simulink model "state_machine_by_cod_1_sm_master"  (R2021b)
settings: Solver=ode4  StartTime=0.0  StopTime=inf  FixedStep=0.001  RelTol=1e-3  EnableMultiTasking=on
model workspace (MATLAB code in the model file):
  | addpath src\model
  | addpath src\utils
libraries: opal_lib x3
Description:
  | Model of a simple control system for use iin training.
settings Model: Creator=Paul Baracos  LastModifiedBy=andrerangel
settings SolverCC: AlgebraicLoopSolver=TrustRegion
settings DataIOCC: LimitDataPoints=on  SaveFormat=Array  SignalLoggingSaveFormat=ModelDataLogs  SaveOutput=off  SaveTime=off  ReturnWorkspaceOutputs=off  SignalLoggingName=sigsOut
settings OptimizationCC: BlockReduction=off  BooleanDataType=off  OptimizeBlockIOStorage=off  BufferReuse=off  ExpressionFolding=off  LocalBlockOutputs=off  InitFltsAndDblsToZero=on  LifeSpan=inf
settings DebuggingCC: SaveWithParameterizedLinksMsg=none  UnderspecifiedInitializationDetection=Classic  MergeDetectMultiDrivingBlocksExec=none  SignalResolutionControl=TryResolveAllWithWarning  MultiTaskDSMMsg=warning  MultiTaskCondExecSysMsg=none  FcnCallInpInsideContextMsg=warning  SFUnexpectedBacktrackingDiag=warning  SFNoUnconditionalDefaultTransitionDiag=warning  SFExecutionAtInitializationDiag=none  SFMachineParentedDataDiag=warning  ArithmeticOperatorsInVariantConditions=warning
settings HardwareCC: ProdBitPerPointer=32  ProdBitPerSizeT=32  ProdBitPerPtrDiffT=32  ProdLargestAtomicFloat=None  ProdIntDivRoundTo=Undefined  ProdEndianess=Unspecified  ProdWordSize=32  ProdHWDeviceType=32-bit Generic  TargetUnknown=on
settings ModelReferenceCC: PropagateSignalLabelsOutOfModel=off
settings SFSimCC: SimUseLocalCustomCode=off  CustomCodeUndefinedFunction=UseInterfaceOnly
settings RTWCC: GenCodeOnly=on  RTWUseLocalCustomCode=off
settings CodeAppCC: StateflowObjectComments=on
settings GRTTargetCC: TargetFcnLib=ansi_tfl_tmw.mat  TargetLangStandard=C89/C90 (ANSI)  CombineOutputUpdateFcns=off  GRTInterface=on
settings ConfigComp: CovMetricSettings=dw  CovSaveCumulativeToWorkspaceVar=on  CovSaveSingleToWorkspaceVar=on  CovExternalEMLEnable=off

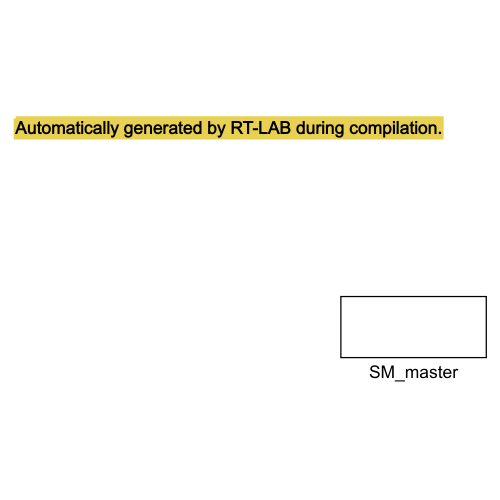
[thumbnail: Simulink's stored preview of the top-level diagram]
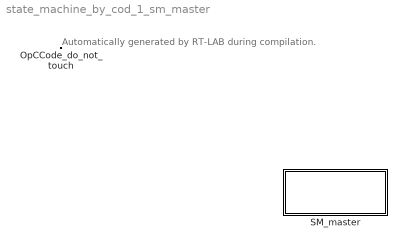
== system state_machine_by_cod_1_sm_master ==
  note: Automatically generated by RT-LAB during compilation.
  OpCCode_do_not_touch : opal_lib/Communication/OpCCode  SystemSampleTime=-1  VariantActivationTime=update diagram  Latency=0  AutoFrameSizeCalculation=off
  SM_master : Subsystem

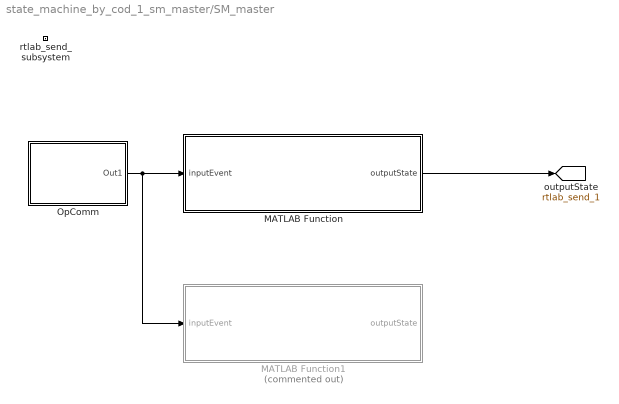
== system state_machine_by_cod_1_sm_master/SM_master ==
  MATLAB Function : MATLAB Function  TreatAsAtomicUnit=on
  MATLAB Function1 : MATLAB Function  Commented=on  TreatAsAtomicUnit=on
  OpComm : Subsystem
      mask init:
      | opmaskdisplay('maskdisplay_block',gcb,'disp(''OpComm'')');
      mask Display:
      | patch([0 0.5 0.7 0],[1 1 0 0],[0.7 0.75 0.9]);
      | patch([1 0.53 0.73 1],[1 1 0 0],[1 0.8 0.7]);
      | plot([0 0 1 1 0],[0 1 1 0 0]);
      | disp('OpComm')
  rtlab_send_subsystem : Subsystem  Priority=-100
      mask Display: text(0,0,'');
  tag scope: rtlab_send_1=global
  wires:
  MATLAB Function/1(outputState) -> [rtlab_send_1]
  OpComm/1(Out1) -> MATLAB Function1/1(inputEvent), MATLAB Function/1(inputEvent)

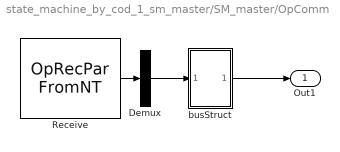
== system state_machine_by_cod_1_sm_master/SM_master/OpComm ==
  Demux : Demux  Outputs=[1]
  Receive : opal_lib/Communication/OpRecPar FromNT  Data_width=1  InitialConditions=3
  busStruct : Subsystem
  Out1 : Outport
  wires:
  Demux/1 -> busStruct/1(In1)
  busStruct/1(Out1) -> Out1/1
  Receive/1 -> Demux/1

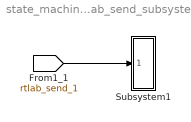
== system state_machine_by_cod_1_sm_master/SM_master/rtlab_send_subsystem ==
  Subsystem1 : Subsystem
  wires:
  [rtlab_send_1] -> Subsystem1/1(In1)

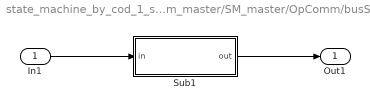
== system state_machine_by_cod_1_sm_master/SM_master/OpComm/busStruct ==
  In1 : Inport
  Sub1 : Subsystem
  Out1 : Outport
  wires:
  Sub1/1(out) -> Out1/1
  In1/1 -> Sub1/1(in)

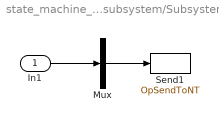
== system state_machine_by_cod_1_sm_master/SM_master/rtlab_send_subsystem/Subsystem1 ==
  In1 : Inport
  Mux : Mux  Inputs=1
  Send1 : opal_lib/Communication/OpSendToNT  Acqu_group=1
  wires:
  Mux/1 -> Send1/1
  In1/1 -> Mux/1

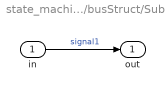
== system state_machine_by_cod_1_sm_master/SM_master/OpComm/busStruct/Sub1 ==
  in : Inport
  out : Outport
  wires:
  in/1 -> out/1  "signal1"

== matlab function state_machine_by_cod_1_sm_master/SM_master/MATLAB Function ==
  data: inputEvent input; outputState output size=[1 1]
function outputState   = stateMachineFcn(inputEvent)
% Example of a State Machine with 3 states.
persistent stateMachine

if (isempty(stateMachine))
    
    % Create the states with the State Class.
    s0 = State(0, 's0', [1,0,1,1,1]);
    s1 = State(1, 's1', [1,1,0,1,1]);
    s2 = State(2, 's2', [1,0,1,1,1]);

    % Group it in a cell array.
    statesArray = {s0, s1, s2};

    % Transitions matrix where each line represents a transition: 
    % event 2 makes a transitions from state 0 to 2 is represented as 
    % [0 2 1]
    transitions = [0, 1 0; 0, 2, 1; 1, 3, 0; 1, 4, 2; 2, 5, 1; 2, 1, 0];

    % Array with the number of the events.
    eventsArray = [1 2 3 4 5];
    stateMachine = StateMachine(statesArray, transitions, eventsArray);
end

stateMachine.inputEvent = inputEvent;
outputState = double(stateMachine.currentState.number);

%activeEvents = stateMachine.currentState.activeEvents;

== matlab function state_machine_by_cod_1_sm_master/SM_master/MATLAB Function1 ==
  data: inputEvent input; outputState output size=[1 1]
function outputState   = stateMachineDebug(inputEvent)
% Example of a State Machine with 3 states.
persistent stateMachine
persistent statesArray
persistent transitions
persistent stateNumber
persistent stateIndex
persistent numberOfStates
persistent eventsArray

if (isempty(stateMachine))
    stateMachine = 1;
    % Create the states with the State Class.
    s0 = State(0, 's0', [1,0,1,1,1]);
    s1 = State(1, 's1', [1,1,0,1,1]);
    s2 = State(2, 's2', [1,0,1,1,1]);

    % Group it in a cell array.
    statesArray = {s0, s1, s2};

    % Transitions matrix where each line represents a transition: 
    % event 2 makes a transitions from state 0 to 2 is represented as 
    % [0 2 1]
    transitions = [0, 1 0; 0, 2, 1; 1, 3, 0; 1, 4, 2; 2, 5, 1; 2, 1, 0];

    % Array with the number of the events.
    eventsArray = [1 2 3 4 5];
    %stateMachine = StateMachine(statesArray, transitions, eventsArray);
    numberOfStates = length(statesArray);
    
    % Default state as the first.
    stateNumber = statesArray{1}.number;
    stateIndex = 1;
end

% Set the input event.
%stateMachine.inputEvent = inputEvent;

% Get the output state.
outputState = stateMachine.currentState.number;

%activeEvents = stateMachine.currentState.activeEvents;
